simulink model "stackerPositioning_tIB"  (R2014b)
settings: Solver=FixedStepDiscrete  StartTime=0.0  StopTime=10.0  RelTol=1e-3
libraries: c2833xlib x3, c280xlib x1
settings Model: Creator=Michael  LastModifiedBy=Michael
settings DataIOCC: SaveOutput=off  SaveTime=off
settings OptimizationCC: OptimizeModelRefInitCode=on  LifeSpan=1
settings HardwareCC: ProdBitPerChar=16  ProdBitPerInt=16  ProdBitPerPointer=16  ProdLargestAtomicInteger=Integer  ProdIntDivRoundTo=Zero  ProdEndianess=LittleEndian  ProdWordSize=16  ProdHWDeviceType=Texas Instruments->C2000
settings RTWCC: SystemTargetFile=idelink_ert.tlc  GenerateMakefile=off  TemplateMakefile=none  Description=IDE Link ERT  ProcessScript=idelink_ert_make_rtw_hook  Toolchain=Texas Instruments Code Composer Studio v5 (C2000)
settings CodeAppCC: IgnoreCustomStorageClasses=off
settings TargetHardwareResources: Description=Target Hardware Resources Component

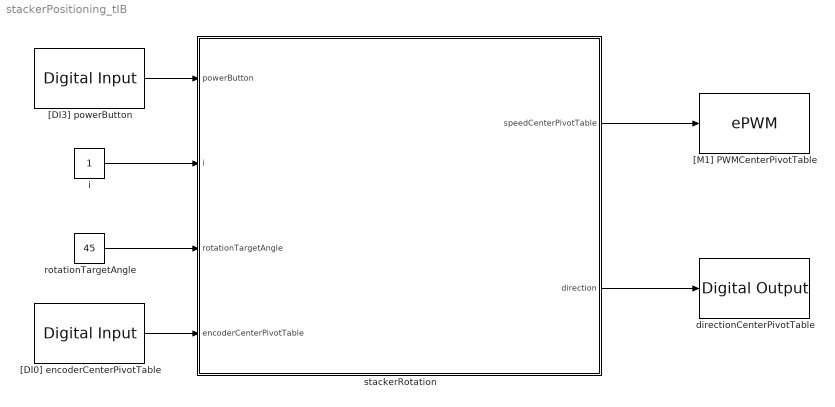
== system stackerPositioning_tIB ==
  "[DI0] encoderCenterPivotTable" : c2833xlib/Digital Input  GPIO_Number=GPIO24~GPIO31  GPIO_Bit0=on  GPIO_Bit1=off  GPIO_Bit2=off  GPIO_Bit3=off  GPIO_Bit4=off  GPIO_Bit5=off  GPIO_Bit6=off  GPIO_Bit7=off  sampleTime=0.001  dataType=boolean  GPIO_Bit0_Qualification=Sync to SYSCLKOUT  GPIO_Bit1_Qualification=Sync to SYSCLKOUT  GPIO_Bit2_Qualification=Sync to SYSCLKOUT  GPIO_Bit3_Qualification=Sync to SYSCLKOUT  GPIO_Bit4_Qualification=Sync to SYSCLKOUT  GPIO_Bit5_Qualification=Sync to SYSCLKOUT  GPIO_Bit6_Qualification=Sync to SYSCLKOUT  GPIO_Bit7_Qualification=Sync to SYSCLKOUT  Qualification_Period=-1
  "[DI3] powerButton" : c2833xlib/Digital Input  GPIO_Number=GPIO32~GPIO39  GPIO_Bit0=off  GPIO_Bit1=on  GPIO_Bit2=off  GPIO_Bit3=off  GPIO_Bit4=off  GPIO_Bit5=off  GPIO_Bit6=off  GPIO_Bit7=off  sampleTime=0.001  dataType=boolean  GPIO_Bit0_Qualification=Sync to SYSCLKOUT  GPIO_Bit1_Qualification=Sync to SYSCLKOUT  GPIO_Bit2_Qualification=Sync to SYSCLKOUT  GPIO_Bit3_Qualification=Sync to SYSCLKOUT  GPIO_Bit4_Qualification=Sync to SYSCLKOUT  GPIO_Bit5_Qualification=Sync to SYSCLKOUT  GPIO_Bit6_Qualification=Sync to SYSCLKOUT  GPIO_Bit7_Qualification=Sync to SYSCLKOUT  Qualification_Period=-1
  "[M1] PWMCenterPivotTable" : c280xlib/ePWM  checkMode=off  useModule=ePWM2  periodUnits=Clock cycles  timerSource=Specify via dialog  timerPeriod_clk=64000  timerPeriod_sec=0.0001  tbshadow=Counter equals to zero  countingMode=Up  phaseActiveEnable=Disable  phaseDirection=Count down after sync  phaseActive=0  synchronizationEnable=off  synchronizationOption=Disable  clockPrescale=1  HSclockPrescale=1  ePWMxAStatus=off  CMPAUnits=Clock cycles  CMPASource=Specify via dialog  CMPAValue_per=50  CMPAValue_clk=32000  enCMPAshadow=Counter equals to zero  ePWMxAactionLogic1=Do nothing  ePWMxAactionLogic2=Clear  ePWMxAactionLogic3=Set  ePWMxAactionLogic4=Do nothing  ePWMxAactionLogic5=Do nothing  ePWMxAactionLogic6=Do nothing  ePWMxALoadMode=Load on counter equals to zero (CTR=Zero)  ePWMxACSFenable=off  ePWMxACSFvalue=Forcing disable  ePWMxASFreload=Zero  enHRPWM=off  HRPWM_LoadMode=Counter equals to zero (CTR=ZERO)  HRPWM_CTLMode=Phase control mode  HRPWM_EDGMode=Both edge  enSFO=on  ePWMxBStatus=on  CMPBUnits=Percentages  CMPBSource=Input port  CMPBValue_per=35  CMPBValue_clk=32000  enCMPBshadow=Counter equals to zero  ePWMxBactionLogic1=Do nothing  ePWMxBactionLogic2=Set  ePWMxBactionLogic3=Do nothing  ePWMxBactionLogic4=Do nothing  ePWMxBactionLogic5=Clear  ePWMxBactionLogic6=Do nothing  ePWMxBLoadMode=Load on counter equals to zero (CTR=Zero)  ePWMxBCSFenable=off  ePWMxBCSFvalue=Forcing disable  ePWMxBSFreload=Zero  enableDBePWMxA=off  enableDBePWMxB=off  DBpolarity=Active high (AH)  DBedgeDelay=Positive  DBSource_ePWMxA=ePWMxA  DBSource_ePWMxB=ePWMxA  DBperiodSource=Specify via dialog  REDperiod=0  FEDperiod=0  adcstartModuleA=off  adcrequestEventA=First event  adcstartEventA=Counter equals to zero (CTR=Zero)  adcstartModuleB=off  adcrequestEventB=First event  adcstartEventB=Counter equals to zero (CTR=Zero)  intEn=off  intPrd=First event  intSel=Counter equals to zero (CTR=Zero)  chopperEnable=off  chopperFrequency=1  chopperFirstwidth=1  chopperDuty=12.5%  tripZonesource=Specify via dialog  tzselOSHT1=off  tzselOSHT2=off  tzselOSHT3=off  tzselOSHT4=off  tzselOSHT5=off  tzselOSHT6=off  tzselCBC1=off  tzselCBC2=off  tzselCBC3=off  tzselCBC4=off  tzselCBC5=off  tzselCBC6=off  enTzOstIntr=off  enTzCbcIntr=off  ePWMxAforced=No action  ePWMxBforced=No action  timerPeriod=-1  ePWMxAValue=0  ePWMxBValue=0  tripZoneoption=One-shot trip (OSHT)
  directionCenterPivotTable : c2833xlib/Digital Output  GPIO_Number=GPIO16~GPIO23  GPIO_Bit0=off  GPIO_BIT0_Toggle=off  GPIO_Bit1=off  GPIO_BIT1_Toggle=off  GPIO_Bit2=off  GPIO_BIT2_Toggle=off  GPIO_Bit3=off  GPIO_BIT3_Toggle=off  GPIO_Bit4=off  GPIO_BIT4_Toggle=off  GPIO_Bit5=on  GPIO_BIT5_Toggle=off  GPIO_Bit6=off  GPIO_BIT6_Toggle=off  GPIO_Bit7=off  GPIO_BIT7_Toggle=off
  i : Constant  OutDataTypeStr=single
  rotationTargetAngle : Constant  Value=45  OutDataTypeStr=single
  stackerRotation : Stateflow chart  TreatAsAtomicUnit=on
  wires:
  i/1 -> stackerRotation/2(i)
  rotationTargetAngle/1 -> stackerRotation/3(rotationTargetAngle)
  stackerRotation/1(speedCenterPivotTable) -> "[M1] PWMCenterPivotTable"/1
  stackerRotation/2(direction) -> directionCenterPivotTable/1
  "[DI0] encoderCenterPivotTable"/1 -> stackerRotation/4(encoderCenterPivotTable)
  "[DI3] powerButton"/1 -> stackerRotation/1(powerButton)

== stateflow chart stackerPositioning_tIB/stackerRotation ==
  state stackerRotation [parallel]
    settings: executionOrder=1
    state start
      entry: direction = [rotationTargetAngle >= 0];
      speedCenterPivotTable = uint16(0);
      targetTics = abs(rotationTargetAngle/360*75*i);
    state waitingForStart
    state targetAngleReached
      entry: speedCenterPivotTable = uint16(0);
    state move
      entry: speedCenterPivotTable = uint16(100);
    (default) -> waitingForStart : [powerButton == true]
    waitingForStart -> stackerRotation.start : [powerButton == false]
    stackerRotation.start -> move : {send(counterRotation.RESET)}
    move -> targetAngleReached : [counterRotation.count >= targetTics]
  state counterRotation [parallel]
    settings: executionOrder=2
    state start
      entry: count= uint32(0);
    state highLevel
    state lowLevel
      entry: count = count + 1;
    lowLevel -> highLevel : [encoderCenterPivotTable > 0]
    (default) -> counterRotation.start
    counterRotation.start -> lowLevel : [encoderCenterPivotTable > 0]
    highLevel -> lowLevel : [encoderCenterPivotTable == 0]
    counterRotation -> counterRotation.start : RESET
  data: targetTics local single [0..]; count local uint32; powerButton input; i input single [0..]; speedCenterPivotTable output uint16 [0..100]; direction output boolean; rotationTargetAngle input single [-360..360]; encoderCenterPivotTable input boolean
  data i settings: description=transition ration of the stacker center pivot plate
  data speedCenterPivotTable settings: description=speedCenterPivotTable of the center pivot table motor
  data direction settings: description=direciton of the center pivot table motor
  data rotationTargetAngle settings: description=rotation target angle for the center pivot table of the stacker
  data encoderCenterPivotTable settings: description=encoder signal of the center pivot table motor
  events: RESET local FUNCTION_CALL_EVENT
